simulink model "MicrochipTargetMotorControl"  (R2024b)
settings: Solver=FixedStepDiscrete  StartTime=0.0  StopTime=50  RelTol=1e-3  EnableMultiTasking=on
InitFcn:
  | MicrochipTargetMotorControlData;
  | mcbMotorSwapData;
values from neighbouring files (symbols this model uses):
  Ts = T_pwm    [mcbMotorSwapData.m]
  Ts_motor = T_pwm/2    [mcbMotorSwapData.m]
  Ts_serialIn = 50e-3    (= 0.05)    [MicrochipTargetMotorControlData.m]
  Ts_speed = 10*Ts    [mcbMotorSwapData.m]
undefined symbols (not defined in the file or in its folder): A4, B0, C10, C11, C6, C7, C8, inverter, MaxPer, P17, P20, P39, P40, P41, P43, P44, Pin, pmsm, Resol, s, target, Timer, us
libraries: MCHP_Blockset x19, simulink x13, autolibpmsminterior x1, mcbplantlib x1, mcbcontrolslib x1
(part 3 of 4)

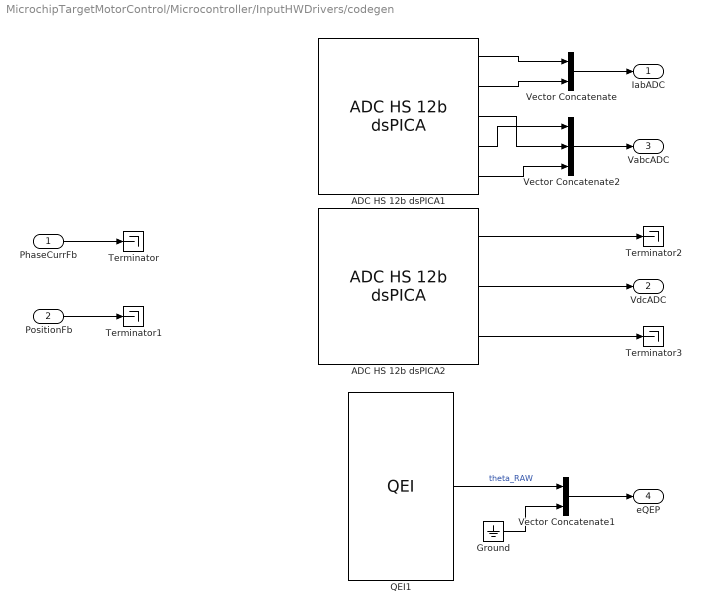
== system MicrochipTargetMotorControl/Microcontroller/InputHWDrivers/codegen ==
  PhaseCurrFb : Inport
  PositionFb : Inport  Port=2
  ADC HS 12b dsPICA1 : MCHP_Blockset/Analog IO/ADC HS 12b dsPICA  ADCREF=ADC 1 and ADC 2  ADC1_refChannel=0 (highest priority)  ADC2_refChannel=0 (highest priority)  ADC3_refChannel=Not used  ADC4_refChannel=Not used  ADC5_refChannel=Not used  CALRATE=once at startup  VREF_RNG=3.0V to 3.6V  BUFEN=off  info=0  SampleTime=Ts  MCHP_PORT={ADC1_seq0.0}{ADC1A2}15:2:A2;{ADC2_seq0.0}{ADC2B0}15:2:B0;{ADC1_seq0.1}{ADC1B8}15:2:B8;{ADC2_seq0.1}{ADC2B9}15:2:B9;{ADC2_seq0.2}{ADC2A10}15:2:A10;{ADC1_seq0.0}{ADC1A2}15:2:A2;{ADC2_seq0.0}{ADC2B0}15:2:B0;{ADC1_seq0.1}{ADC1B8}15:2:B8;{ADC2_seq0.1}{ADC2B9}15:2:B9;{ADC2_seq0.2}{ADC2A10}15:2:A10;  MCHP_MASTERLINK=MicrochipTargetMotorControl/Microcontroller/HWConfigurations/Microchip Master  MCHP_CRC=34200121  ADC_Synchronisation=Triggered by custom source  ADC_Trig_TXT=PWM1_Trg1  ADC_TrigTimeStep=on  TrigSource_seq0_TXT=PWM1 adc trig 0  SampleTime_seq0_Tad_TXT="4.5 Tad  = 56.2ns  -  Rin < 5.2 kOhm"  ADC1_seq0_TXT=AD1 AN0 / A2 / Pin[12]  ADC1_seq0_align=Right aligned  ADC1_seq0_overSampling=x1 (12 bits)  ADC2_seq0_TXT=AD2 AN1 / B0 / Pin[20]  ADC2_seq0_align=Right aligned  ADC2_seq0_overSampling=x1 (12 bits)  ADC3_seq0_TXT="AD2 AN1 / B0 / Pin[20]  (L)"  ADC3_seq0_align=Right aligned  ADC3_seq0_overSampling=x1 (12 bits)  ADC4_seq0_TXT="AD2 AN1 / B0 / Pin[20]  (L)"  ADC4_seq0_align=Right aligned  ADC4_seq0_overSampling=x1 (12 bits)  ADC5_seq0_TXT="AD2 AN1 / B0 / Pin[20]  (L)"  ADC5_seq0_align=Right aligned  ADC5_seq0_overSampling=x1 (12 bits)  ADC1_seq0_1_TXT=AD1 AN11 / B8 / Pin[23]  ADC1_seq0_1_align=Right aligned  ADC1_seq0_1_overSampling=x1 (12 bits)  ADC2_seq0_1_TXT=AD2 AN10 / B9 / Pin[24]  ADC2_seq0_1_align=Right aligned  ADC2_seq0_1_overSampling=x1 (12 bits)  ADC3_seq0_1_TXT=Not Used  ADC3_seq0_1_align=Right aligned  ADC3_seq0_1_overSampling=x1 (12 bits)  ADC4_seq0_1_TXT=Not Used  ADC4_seq0_1_align=Right aligned  ADC4_seq0_1_overSampling=x1 (12 bits)  ADC5_seq0_1_TXT=Not Used  ADC5_seq0_1_align=Right aligned  ADC5_seq0_1_overSampling=x1 (12 bits)  ADC1_seq0_2_TXT=Not Used  ADC1_seq0_2_align=Right aligned  ADC1_seq0_2_overSampling=x1 (12 bits)  ADC2_seq0_2_TXT=AD2 AN7 / A10 / Pin[9]  ADC2_seq0_2_align=Right aligned  ADC2_seq0_2_overSampling=x1 (12 bits)  ADC3_seq0_2_TXT=Not Used  ADC3_seq0_2_align=Right aligned  ADC3_seq0_2_overSampling=x1 (12 bits)  ADC4_seq0_2_TXT=Not Used  ADC4_seq0_2_align=Right aligned  ADC4_seq0_2_overSampling=x1 (12 bits)  ADC5_seq0_2_TXT=Not Used  ADC5_seq0_2_align=Right aligned  ADC5_seq0_2_overSampling=x1 (12 bits)  ADC1_seq0_3_TXT=Not Used  ADC1_seq0_3_align=Right aligned  ADC1_seq0_3_overSampling=x1 (12 bits)  ADC2_seq0_3_TXT=Not Used  ADC2_seq0_3_align=Right aligned  ADC2_seq0_3_overSampling=x1 (12 bits)  ADC3_seq0_3_TXT=Not Used  ADC3_seq0_3_align=Right aligned  ADC3_seq0_3_overSampling=x1 (12 bits)  ADC4_seq0_3_TXT=Not Used  ADC4_seq0_3_align=Right aligned  ADC4_seq0_3_overSampling=x1 (12 bits)  ADC5_seq0_3_TXT=Not Used  ADC5_seq0_3_align=Right aligned  ADC5_seq0_3_overSampling=x1 (12 bits)  ADC1_seq0_4_TXT=Not Used  ADC1_seq0_4_align=Right aligned  ADC1_seq0_4_overSampling=x1 (12 bits)  ADC2_seq0_4_TXT=Not Used  ADC2_seq0_4_align=Right aligned  ADC2_seq0_4_overSampling=x1 (12 bits)  ADC3_seq0_4_TXT=Not Used  ADC3_seq0_4_align=Right aligned  ADC3_seq0_4_overSampling=x1 (12 bits)  ADC4_seq0_4_TXT=Not Used  ADC4_seq0_4_align=Right aligned  ADC4_seq0_4_overSampling=x1 (12 bits)  ADC5_seq0_4_TXT=Not Used  ADC5_seq0_4_align=Right aligned  ADC5_seq0_4_overSampling=x1 (12 bits)  ADC1_seq0_5_TXT=Not Used  ADC1_seq0_5_align=Right aligned  ADC1_seq0_5_overSampling=x1 (12 bits)  ADC2_seq0_5_TXT=Not Used  ADC2_seq0_5_align=Right aligned  ADC2_seq0_5_overSampling=x1 (12 bits)  ADC3_seq0_5_TXT=Not Used  ADC3_seq0_5_align=Right aligned  ADC3_seq0_5_overSampling=x1 (12 bits)  ADC4_seq0_5_TXT=Not Used  ADC4_seq0_5_align=Right aligned  ADC4_seq0_5_overSampling=x1 (12 bits)  ADC5_seq0_5_TXT=Not Used  ADC5_seq0_5_align=Right aligned  ADC5_seq0_5_overSampling=x1 (12 bits)  ADC_TRG2_ACCBRST_seq0=Burst - not interruptible  ADC1_NINSEL_seq0_TXT=Vss - single ended (unsigned)  ADC2_NINSEL_seq0_TXT=Vss - single ended (unsigned)  ADC3_NINSEL_seq0_TXT=Vss - single ended (unsigned)  ADC4_NINSEL_seq0_TXT=Vss - single ended (unsigned)  ADC5_NINSEL_seq0_TXT=Vss - single ended (unsigned)  TrigTimeStep_seq0=on  info_seq0=0  TrigSource_seq1_TXT=after previous sequence  SampleTime_seq1_Tad_TXT="0.5 Tad  = 6.25ns  -  Rin < 0 kOhm"  ADC1_seq1_TXT=Not Used  ADC1_seq1_align=Right aligned  ADC1_seq1_overSampling=x1 (12 bits)  ADC2_seq1_TXT=Not Used  ADC2_seq1_align=Right aligned  ADC2_seq1_overSampling=x1 (12 bits)  ADC3_seq1_TXT=Not Used  ADC3_seq1_align=Right aligned  ADC3_seq1_overSampling=x1 (12 bits)  ADC4_seq1_TXT=Not Used  ADC4_seq1_align=Right aligned  ADC4_seq1_overSampling=x1 (12 bits)  ADC5_seq1_TXT=Not Used  ADC5_seq1_align=Right aligned  ADC5_seq1_overSampling=x1 (12 bits)  ADC1_seq1_1_TXT=Not Used  ADC1_seq1_1_align=Right aligned  ADC1_seq1_1_overSampling=x1 (12 bits)  ADC2_seq1_1_TXT=Not Used  ADC2_seq1_1_align=Right aligned  ADC2_seq1_1_overSampling=x1 (12 bits)  ADC3_seq1_1_TXT=Not Used  ADC3_seq1_1_align=Right aligned  ADC3_seq1_1_overSampling=x1 (12 bits)  ADC4_seq1_1_TXT=Not Used  ADC4_seq1_1_align=Right aligned  ADC4_seq1_1_overSampling=x1 (12 bits)  ADC5_seq1_1_TXT=Not Used  ADC5_seq1_1_align=Right aligned  ADC5_seq1_1_overSampling=x1 (12 bits)  ADC1_seq1_2_TXT=Not Used  ADC1_seq1_2_align=Right aligned  ADC1_seq1_2_overSampling=x1 (12 bits)  ADC2_seq1_2_TXT=Not Used  ADC2_seq1_2_align=Right aligned  ADC2_seq1_2_overSampling=x1 (12 bits)  ADC3_seq1_2_TXT=Not Used  ADC3_seq1_2_align=Right aligned  ADC3_seq1_2_overSampling=x1 (12 bits)  ADC4_seq1_2_TXT=Not Used  ADC4_seq1_2_align=Right aligned  ADC4_seq1_2_overSampling=x1 (12 bits)  ADC5_seq1_2_TXT=Not Used  ADC5_seq1_2_align=Right aligned  ADC5_seq1_2_overSampling=x1 (12 bits)  ADC1_seq1_3_TXT=Not Used  ADC1_seq1_3_align=Right aligned  ADC1_seq1_3_overSampling=x1 (12 bits)  ADC2_seq1_3_TXT=Not Used  ADC2_seq1_3_align=Right aligned  ADC2_seq1_3_overSampling=x1 (12 bits)  ADC3_seq1_3_TXT=Not Used  ADC3_seq1_3_align=Right aligned  ADC3_seq1_3_overSampling=x1 (12 bits)  ADC4_seq1_3_TXT=Not Used  ADC4_seq1_3_align=Right aligned  ADC4_seq1_3_overSampling=x1 (12 bits)  ADC5_seq1_3_TXT=Not Used  ADC5_seq1_3_align=Right aligned  ADC5_seq1_3_overSampling=x1 (12 bits)  ADC1_seq1_4_TXT=Not Used  ADC1_seq1_4_align=Right aligned  ADC1_seq1_4_overSampling=x1 (12 bits)  ADC2_seq1_4_TXT=Not Used  ADC2_seq1_4_align=Right aligned  ADC2_seq1_4_overSampling=x1 (12 bits)  ADC3_seq1_4_TXT=Not Used  ADC3_seq1_4_align=Right aligned  ADC3_seq1_4_overSampling=x1 (12 bits)  ADC4_seq1_4_TXT=Not Used  ADC4_seq1_4_align=Right aligned  ADC4_seq1_4_overSampling=x1 (12 bits)  ADC5_seq1_4_TXT=Not Used  ADC5_seq1_4_align=Right aligned  ADC5_seq1_4_overSampling=x1 (12 bits)  ADC1_seq1_5_TXT=Not Used  ADC1_seq1_5_align=Right aligned  ADC1_seq1_5_overSampling=x1 (12 bits)  ADC2_seq1_5_TXT=Not Used  ADC2_seq1_5_align=Right aligned  ADC2_seq1_5_overSampling=x1 (12 bits)  ADC3_seq1_5_TXT=Not Used  ADC3_seq1_5_align=Right aligned  ADC3_seq1_5_overSampling=x1 (12 bits)  ADC4_seq1_5_TXT=Not Used  ADC4_seq1_5_align=Right aligned  ADC4_seq1_5_overSampling=x1 (12 bits)  ADC5_seq1_5_TXT=Not Used  ADC5_seq1_5_align=Right aligned  ADC5_seq1_5_overSampling=x1 (12 bits)  ADC_TRG2_ACCBRST_seq1=Burst - not interruptible  ADC1_NINSEL_seq1_TXT=Vss - single ended (unsigned)  ADC2_NINSEL_seq1_TXT=Vss - single ended (unsigned)  ADC3_NINSEL_seq1_TXT=Vss - single ended (unsigned)  ADC4_NINSEL_seq1_TXT=Vss - single ended (unsigned)  ADC5_NINSEL_seq1_TXT=Vss - single ended (unsigned)  TrigTimeStep_seq1=off  info_seq1=0  TrigSource_seq2_TXT=after previous sequence  SampleTime_seq2_Tad_TXT="0.5 Tad  = 6.25ns  -  Rin < 0 kOhm"  ADC1_seq2_TXT=Not Used  ADC1_seq2_align=Right aligned  ADC1_seq2_overSampling=x1 (12 bits)  ADC2_seq2_TXT=Not Used  ADC2_seq2_align=Right aligned  ADC2_seq2_overSampling=x1 (12 bits)  ADC3_seq2_TXT=Not Used  ADC3_seq2_align=Right aligned  ADC3_seq2_overSampling=x1 (12 bits)  ADC4_seq2_TXT=Not Used  ADC4_seq2_align=Right aligned  ADC4_seq2_overSampling=x1 (12 bits)  ADC5_seq2_TXT=Not Used  ADC5_seq2_align=Right aligned  ADC5_seq2_overSampling=x1 (12 bits)  ADC1_seq2_1_TXT=Not Used  ADC1_seq2_1_align=Right aligned  ADC1_seq2_1_overSampling=x1 (12 bits)  ADC2_seq2_1_TXT=Not Used  ADC2_seq2_1_align=Right aligned  ADC2_seq2_1_overSampling=x1 (12 bits)  ADC3_seq2_1_TXT=Not Used  ADC3_seq2_1_align=Right aligned  ADC3_seq2_1_overSampling=x1 (12 bits)  ADC4_seq2_1_TXT=Not Used  ADC4_seq2_1_align=Right aligned  ADC4_seq2_1_overSampling=x1 (12 bits)  ADC5_seq2_1_TXT=Not Used  ADC5_seq2_1_align=Right aligned  ADC5_seq2_1_overSampling=x1 (12 bits)  ADC1_seq2_2_TXT=Not Used  ADC1_seq2_2_align=Right aligned  ADC1_seq2_2_overSampling=x1 (12 bits)  ADC2_seq2_2_TXT=Not Used  ADC2_seq2_2_align=Right aligned  ADC2_seq2_2_overSampling=x1 (12 bits)  ADC3_seq2_2_TXT=Not Used  ADC3_seq2_2_align=Right aligned  ADC3_seq2_2_overSampling=x1 (12 bits)  ADC4_seq2_2_TXT=Not Used  ADC4_seq2_2_align=Right aligned  ADC4_seq2_2_overSampling=x1 (12 bits)  ADC5_seq2_2_TXT=Not Used  ADC5_seq2_2_align=Right aligned  ADC5_seq2_2_overSampling=x1 (12 bits)  ADC1_seq2_3_TXT=Not Used  ADC1_seq2_3_align=Right aligned  ADC1_seq2_3_overSampling=x1 (12 bits)  ADC2_seq2_3_TXT=Not Used  ADC2_seq2_3_align=Right aligned  ADC2_seq2_3_overSampling=x1 (12 bits)  ADC3_seq2_3_TXT=Not Used  ADC3_seq2_3_align=Right aligned  ADC3_seq2_3_overSampling=x1 (12 bits)  ADC4_seq2_3_TXT=Not Used  ADC4_seq2_3_align=Right aligned  ADC4_seq2_3_overSampling=x1 (12 bits)  ADC5_seq2_3_TXT=Not Used  ADC5_seq2_3_align=Right aligned  ADC5_seq2_3_overSampling=x1 (12 bits)  ADC1_seq2_4_TXT=Not Used  ADC1_seq2_4_align=Right aligned  ADC1_seq2_4_overSampling=x1 (12 bits)  ADC2_seq2_4_TXT=Not Used  ADC2_seq2_4_align=Right aligned  ADC2_seq2_4_overSampling=x1 (12 bits)  ADC3_seq2_4_TXT=Not Used  ADC3_seq2_4_align=Right aligned  ADC3_seq2_4_overSampling=x1 (12 bits)  ADC4_seq2_4_TXT=Not Used  ADC4_seq2_4_align=Right aligned  ADC4_seq2_4_overSampling=x1 (12 bits)  ADC5_seq2_4_TXT=Not Used  ADC5_seq2_4_align=Right aligned  ADC5_seq2_4_overSampling=x1 (12 bits)  ADC1_seq2_5_TXT=Not Used  ADC1_seq2_5_align=Right aligned  ADC1_seq2_5_overSampling=x1 (12 bits)  ADC2_seq2_5_TXT=Not Used  ADC2_seq2_5_align=Right aligned  ADC2_seq2_5_overSampling=x1 (12 bits)  ADC3_seq2_5_TXT=Not Used  ADC3_seq2_5_align=Right aligned  ADC3_seq2_5_overSampling=x1 (12 bits)  ADC4_seq2_5_TXT=Not Used  ADC4_seq2_5_align=Right aligned  ADC4_seq2_5_overSampling=x1 (12 bits)  ADC5_seq2_5_TXT=Not Used  ADC5_seq2_5_align=Right aligned  ADC5_seq2_5_overSampling=x1 (12 bits)  ADC_TRG2_ACCBRST_seq2=Burst - not interruptible  ADC1_NINSEL_seq2_TXT=Vss - single ended (unsigned)  ADC2_NINSEL_seq2_TXT=Vss - single ended (unsigned)  ADC3_NINSEL_seq2_TXT=Vss - single ended (unsigned)  ADC4_NINSEL_seq2_TXT=Vss - single ended (unsigned)  ADC5_NINSEL_seq2_TXT=Vss - single ended (unsigned)  TrigTimeStep_seq2=off  info_seq2=0  TrigSource_seq3_TXT=after previous sequence  SampleTime_seq3_Tad_TXT="0.5 Tad  = 6.25ns  -  Rin < 0 kOhm"  ADC1_seq3_TXT=Not Used  ADC1_seq3_align=Right aligned  ADC1_seq3_overSampling=x1 (12 bits)  ADC2_seq3_TXT=Not Used  ADC2_seq3_align=Right aligned  ADC2_seq3_overSampling=x1 (12 bits)  ADC3_seq3_TXT=Not Used  ADC3_seq3_align=Right aligned  ADC3_seq3_overSampling=x1 (12 bits)  ADC4_seq3_TXT=Not Used  ADC4_seq3_align=Right aligned  ADC4_seq3_overSampling=x1 (12 bits)  ADC5_seq3_TXT=Not Used  ADC5_seq3_align=Right aligned  ADC5_seq3_overSampling=x1 (12 bits)  ADC1_seq3_1_TXT=Not Used  ADC1_seq3_1_align=Right aligned  ADC1_seq3_1_overSampling=x1 (12 bits)  ADC2_seq3_1_TXT=Not Used  ADC2_seq3_1_align=Right aligned  ADC2_seq3_1_overSampling=x1 (12 bits)  ADC3_seq3_1_TXT=Not Used  ADC3_seq3_1_align=Right aligned  ADC3_seq3_1_overSampling=x1 (12 bits)  ADC4_seq3_1_TXT=Not Used  ADC4_seq3_1_align=Right aligned  ADC4_seq3_1_overSampling=x1 (12 bits)  ADC5_seq3_1_TXT=Not Used  ADC5_seq3_1_align=Right aligned  ADC5_seq3_1_overSampling=x1 (12 bits)  ADC1_seq3_2_TXT=Not Used  ADC1_seq3_2_align=Right aligned  ADC1_seq3_2_overSampling=x1 (12 bits)  ADC2_seq3_2_TXT=Not Used  ADC2_seq3_2_align=Right aligned  ADC2_seq3_2_overSampling=x1 (12 bits)  ADC3_seq3_2_TXT=Not Used  ADC3_seq3_2_align=Right aligned  ADC3_seq3_2_overSampling=x1 (12 bits)  ADC4_seq3_2_TXT=Not Used  ADC4_seq3_2_align=Right aligned  ADC4_seq3_2_overSampling=x1 (12 bits)  ADC5_seq3_2_TXT=Not Used  ADC5_seq3_2_align=Right aligned  ADC5_seq3_2_overSampling=x1 (12 bits)  ADC1_seq3_3_TXT=Not Used  ADC1_seq3_3_align=Right aligned  ADC1_seq3_3_overSampling=x1 (12 bits)  ADC2_seq3_3_TXT=Not Used  ADC2_seq3_3_align=Right aligned  ADC2_seq3_3_overSampling=x1 (12 bits)  ADC3_seq3_3_TXT=Not Used  ADC3_seq3_3_align=Right aligned  ADC3_seq3_3_overSampling=x1 (12 bits)  ADC4_seq3_3_TXT=Not Used  ADC4_seq3_3_align=Right aligned  ADC4_seq3_3_overSampling=x1 (12 bits)  ADC5_seq3_3_TXT=Not Used  ADC5_seq3_3_align=Right aligned  ADC5_seq3_3_overSampling=x1 (12 bits)  ADC1_seq3_4_TXT=Not Used  ADC1_seq3_4_align=Right aligned  ADC1_seq3_4_overSampling=x1 (12 bits)  ADC2_seq3_4_TXT=Not Used  ADC2_seq3_4_align=Right aligned  ADC2_seq3_4_overSampling=x1 (12 bits)  ADC3_seq3_4_TXT=Not Used  ADC3_seq3_4_align=Right aligned  ADC3_seq3_4_overSampling=x1 (12 bits)  ADC4_seq3_4_TXT=Not Used  ADC4_seq3_4_align=Right aligned  ADC4_seq3_4_overSampling=x1 (12 bits)  ADC5_seq3_4_TXT=Not Used  ADC5_seq3_4_align=Right aligned  ADC5_seq3_4_overSampling=x1 (12 bits)  ADC1_seq3_5_TXT=Not Used  ADC1_seq3_5_align=Right aligned  ADC1_seq3_5_overSampling=x1 (12 bits)  ADC2_seq3_5_TXT=Not Used  ADC2_seq3_5_align=Right aligned  ADC2_seq3_5_overSampling=x1 (12 bits)  ADC3_seq3_5_TXT=Not Used  ADC3_seq3_5_align=Right aligned  ADC3_seq3_5_overSampling=x1 (12 bits)  ADC4_seq3_5_TXT=Not Used  ADC4_seq3_5_align=Right aligned  ADC4_seq3_5_overSampling=x1 (12 bits)  ADC5_seq3_5_TXT=Not Used  ADC5_seq3_5_align=Right aligned  ADC5_seq3_5_overSampling=x1 (12 bits)  ADC_TRG2_ACCBRST_seq3=Burst - not interruptible  ADC1_NINSEL_seq3_TXT=Vss - single ended (unsigned)  ADC2_NINSEL_seq3_TXT=Vss - single ended (unsigned)  ADC3_NINSEL_seq3_TXT=Vss - single ended (unsigned)  ADC4_NINSEL_seq3_TXT=Vss - single ended (unsigned)  ADC5_NINSEL_seq3_TXT=Vss - single ended (unsigned)  TrigTimeStep_seq3=off  info_seq3=0  TrigSource_seq4_TXT=after previous sequence  SampleTime_seq4_Tad_TXT="0.5 Tad  = 6.25ns  -  Rin < 0 kOhm"  ADC1_seq4_TXT=Not Used  ADC1_seq4_align=Right aligned  ADC1_seq4_overSampling=x1 (12 bits)  ADC2_seq4_TXT=Not Used  ADC2_seq4_align=Right aligned  ADC2_seq4_overSampling=x1 (12 bits)  ADC3_seq4_TXT=Not Used  ADC3_seq4_align=Right aligned  ADC3_seq4_overSampling=x1 (12 bits)  ADC4_seq4_TXT=Not Used  ADC4_seq4_align=Right aligned  ADC4_seq4_overSampling=x1 (12 bits)  ADC5_seq4_TXT=Not Used  ADC5_seq4_align=Right aligned  ADC5_seq4_overSampling=x1 (12 bits)  ADC1_seq4_1_TXT=Not Used  ADC1_seq4_1_align=Right aligned  ADC1_seq4_1_overSampling=x1 (12 bits)  ADC2_seq4_1_TXT=Not Used  ADC2_seq4_1_align=Right aligned  ADC2_seq4_1_overSampling=x1 (12 bits)  ADC3_seq4_1_TXT=Not Used  ADC3_seq4_1_align=Right aligned  ADC3_seq4_1_overSampling=x1 (12 bits)  ADC4_seq4_1_TXT=Not Used  ADC4_seq4_1_align=Right aligned  ADC4_seq4_1_overSampling=x1 (12 bits)  ADC5_seq4_1_TXT=Not Used  ADC5_seq4_1_align=Right aligned  ADC5_seq4_1_overSampling=x1 (12 bits)  ADC1_seq4_2_TXT=Not Used  ADC1_seq4_2_align=Right aligned  ADC1_seq4_2_overSampling=x1 (12 bits)  ADC2_seq4_2_TXT=Not Used  ADC2_seq4_2_align=Right aligned  ADC2_seq4_2_overSampling=x1 (12 bits)  ADC3_seq4_2_TXT=Not Used  ADC3_seq4_2_align=Right aligned  ADC3_seq4_2_overSampling=x1 (12 bits)  ADC4_seq4_2_TXT=Not Used  ADC4_seq4_2_align=Right aligned  ADC4_seq4_2_overSampling=x1 (12 bits)  ADC5_seq4_2_TXT=Not Used  ADC5_seq4_2_align=Right aligned  ADC5_seq4_2_overSampling=x1 (12 bits)  ADC1_seq4_3_TXT=Not Used  ADC1_seq4_3_align=Right aligned  ADC1_seq4_3_overSampling=x1 (12 bits)  ADC2_seq4_3_TXT=Not Used  ADC2_seq4_3_align=Right aligned  ADC2_seq4_3_overSampling=x1 (12 bits)  ADC3_seq4_3_TXT=Not Used  ADC3_seq4_3_align=Right aligned  ADC3_seq4_3_overSampling=x1 (12 bits)  ADC4_seq4_3_TXT=Not Used  ADC4_seq4_3_align=Right aligned  ADC4_seq4_3_overSampling=x1 (12 bits)  ADC5_seq4_3_TXT=Not Used  ADC5_seq4_3_align=Right aligned  ADC5_seq4_3_overSampling=x1 (12 bits)  ADC1_seq4_4_TXT=Not Used  ADC1_seq4_4_align=Right aligned  ADC1_seq4_4_overSampling=x1 (12 bits)  ADC2_seq4_4_TXT=Not Used  ADC2_seq4_4_align=Right aligned  ADC2_seq4_4_overSampling=x1 (12 bits)  ADC3_seq4_4_TXT=Not Used  ADC3_seq4_4_align=Right aligned  ADC3_seq4_4_overSampling=x1 (12 bits)  ADC4_seq4_4_TXT=Not Used  ADC4_seq4_4_align=Right aligned  ADC4_seq4_4_overSampling=x1 (12 bits)  ADC5_seq4_4_TXT=Not Used  ADC5_seq4_4_align=Right aligned  ADC5_seq4_4_overSampling=x1 (12 bits)  ADC1_seq4_5_TXT=Not Used  ADC1_seq4_5_align=Right aligned  ADC1_seq4_5_overSampling=x1 (12 bits)  ADC2_seq4_5_TXT=Not Used  ADC2_seq4_5_align=Right aligned  ADC2_seq4_5_overSampling=x1 (12 bits)  ADC3_seq4_5_TXT=Not Used  ADC3_seq4_5_align=Right aligned  ADC3_seq4_5_overSampling=x1 (12 bits)  ADC4_seq4_5_TXT=Not Used  ADC4_seq4_5_align=Right aligned  ADC4_seq4_5_overSampling=x1 (12 bits)  ADC5_seq4_5_TXT=Not Used  ADC5_seq4_5_align=Right aligned  ADC5_seq4_5_overSampling=x1 (12 bits)  ADC_TRG2_ACCBRST_seq4=Burst - not interruptible  ADC1_NINSEL_seq4_TXT=Vss - single ended (unsigned)  ADC2_NINSEL_seq4_TXT=Vss - single ended (unsigned)  ADC3_NINSEL_seq4_TXT=Vss - single ended (unsigned)  ADC4_NINSEL_seq4_TXT=Vss - single ended (unsigned)  ADC5_NINSEL_seq4_TXT=Vss - single ended (unsigned)  TrigTimeStep_seq4=off  info_seq4=0  TrigSource_seq5_TXT=after previous sequence  SampleTime_seq5_Tad_TXT="0.5 Tad  = 6.25ns  -  Rin < 0 kOhm"  ADC1_seq5_TXT=Not Used  ADC1_seq5_align=Right aligned  ADC1_seq5_overSampling=x1 (12 bits)  ADC2_seq5_TXT=Not Used  ADC2_seq5_align=Right aligned  ADC2_seq5_overSampling=x1 (12 bits)  ADC3_seq5_TXT=Not Used  ADC3_seq5_align=Right aligned  ADC3_seq5_overSampling=x1 (12 bits)  ADC4_seq5_TXT=Not Used  ADC4_seq5_align=Right aligned  ADC4_seq5_overSampling=x1 (12 bits)  ADC5_seq5_TXT=Not Used  ADC5_seq5_align=Right aligned  ADC5_seq5_overSampling=x1 (12 bits)  ADC1_seq5_1_TXT=Not Used  ADC1_seq5_1_align=Right aligned  ADC1_seq5_1_overSampling=x1 (12 bits)  ADC2_seq5_1_TXT=Not Used  ADC2_seq5_1_align=Right aligned  ADC2_seq5_1_overSampling=x1 (12 bits)  ADC3_seq5_1_TXT=Not Used  ADC3_seq5_1_align=Right aligned  ADC3_seq5_1_overSampling=x1 (12 bits)  ADC4_seq5_1_TXT=Not Used  ADC4_seq5_1_align=Right aligned  ADC4_seq5_1_overSampling=x1 (12 bits)  ADC5_seq5_1_TXT=Not Used  ADC5_seq5_1_align=Right aligned  ADC5_seq5_1_overSampling=x1 (12 bits)  ADC1_seq5_2_TXT=Not Used  ADC1_seq5_2_align=Right aligned  ADC1_seq5_2_overSampling=x1 (12 bits)  ADC2_seq5_2_TXT=Not Used  ADC2_seq5_2_align=Right aligned  ADC2_seq5_2_overSampling=x1 (12 bits)  ADC3_seq5_2_TXT=Not Used  ADC3_seq5_2_align=Right aligned  ADC3_seq5_2_overSampling=x1 (12 bits)  ADC4_seq5_2_TXT=Not Used  ADC4_seq5_2_align=Right aligned  ADC4_seq5_2_overSampling=x1 (12 bits)  ADC5_seq5_2_TXT=Not Used  ADC5_seq5_2_align=Right aligned  ADC5_seq5_2_overSampling=x1 (12 bits)  ADC1_seq5_3_TXT=Not Used  ADC1_seq5_3_align=Right aligned  ADC1_seq5_3_overSampling=x1 (12 bits)  ADC2_seq5_3_TXT=Not Used  ADC2_seq5_3_align=Right aligned  ADC2_seq5_3_overSampling=x1 (12 bits)  ADC3_seq5_3_TXT=Not Used  ADC3_seq5_3_align=Right aligned  ADC3_seq5_3_overSampling=x1 (12 bits)  ADC4_seq5_3_TXT=Not Used  ADC4_seq5_3_align=Right aligned  ADC4_seq5_3_overSampling=x1 (12 bits)  ADC5_seq5_3_TXT=Not Used  ADC5_seq5_3_align=Right aligned  ADC5_seq5_3_overSampling=x1 (12 bits)  ADC1_seq5_4_TXT=Not Used  ADC1_seq5_4_align=Right aligned  ADC1_seq5_4_overSampling=x1 (12 bits)  ADC2_seq5_4_TXT=Not Used  ADC2_seq5_4_align=Right aligned  ADC2_seq5_4_overSampling=x1 (12 bits)  ADC3_seq5_4_TXT=Not Used  ADC3_seq5_4_align=Right aligned  ADC3_seq5_4_overSampling=x1 (12 bits)  ADC4_seq5_4_TXT=Not Used  ADC4_seq5_4_align=Right aligned  ADC4_seq5_4_overSampling=x1 (12 bits)  ADC5_seq5_4_TXT=Not Used  ADC5_seq5_4_align=Right aligned  ADC5_seq5_4_overSampling=x1 (12 bits)  ADC1_seq5_5_TXT=Not Used  ADC1_seq5_5_align=Right aligned  ADC1_seq5_5_overSampling=x1 (12 bits)  ADC2_seq5_5_TXT=Not Used  ADC2_seq5_5_align=Right aligned  ADC2_seq5_5_overSampling=x1 (12 bits)  ADC3_seq5_5_TXT=Not Used  ADC3_seq5_5_align=Right aligned  ADC3_seq5_5_overSampling=x1 (12 bits)  ADC4_seq5_5_TXT=Not Used  ADC4_seq5_5_align=Right aligned  ADC4_seq5_5_overSampling=x1 (12 bits)  ADC5_seq5_5_TXT=Not Used  ADC5_seq5_5_align=Right aligned  ADC5_seq5_5_overSampling=x1 (12 bits)  ADC_TRG2_ACCBRST_seq5=Burst - not interruptible  ADC1_NINSEL_seq5_TXT=Vss - single ended (unsigned)  ADC2_NINSEL_seq5_TXT=Vss - single ended (unsigned)  ADC3_NINSEL_seq5_TXT=Vss - single ended (unsigned)  ADC4_NINSEL_seq5_TXT=Vss - single ended (unsigned)  ADC5_NINSEL_seq5_TXT=Vss - single ended (unsigned)  TrigTimeStep_seq5=off  info_seq5=0
      settings: SourceProductName=MPLAB Device Blocks for Simulink
  ADC HS 12b dsPICA2 : MCHP_Blockset/Analog IO/ADC HS 12b dsPICA  ADCREF=ADC 1  ADC1_refChannel=5  ADC2_refChannel=5  ADC3_refChannel=Not used  ADC4_refChannel=Not used  ADC5_refChannel=Not used  CALRATE=once at startup  VREF_RNG=3.0V to 3.6V  BUFEN=off  info=0  SampleTime=Ts  MCHP_PORT={ADC1_seq0.0}{ADC1A5}15:2:A5;{ADC1_seq0.1}{ADC1A7}15:2:A7;{ADC1_seq0.2}{ADC1A11}15:2:A11;{ADC1_seq0.0}{ADC1A5}15:2:A5;{ADC1_seq0.1}{ADC1A7}15:2:A7;{ADC1_seq0.2}{ADC1A11}15:2:A11;  MCHP_MASTERLINK=MicrochipTargetMotorControl/Microcontroller/HWConfigurations/Microchip Master  MCHP_CRC=34100181  ADC_Synchronisation=off  ADC_Trig_TXT=off  ADC_TrigTimeStep=off  TrigSource_seq0_TXT=PWM1 adc trig 0  SampleTime_seq0_Tad_TXT="8.5 Tad  = 106ns  -  Rin < 11 kOhm"  ADC1_seq0_TXT=AD1 AN3 / A5 / Pin[15]  ADC1_seq0_align=Right aligned  ADC1_seq0_overSampling=x1 (12 bits)  ADC2_seq0_TXT=Not Used  ADC2_seq0_align=Right aligned  ADC2_seq0_overSampling=x1 (12 bits)  ADC3_seq0_TXT="AD2 AN1 / B0 / Pin[20]  (L)"  ADC3_seq0_align=Right aligned  ADC3_seq0_overSampling=x1 (12 bits)  ADC4_seq0_TXT="AD2 AN1 / B0 / Pin[20]  (L)"  ADC4_seq0_align=Right aligned  ADC4_seq0_overSampling=x1 (12 bits)  ADC5_seq0_TXT="AD2 AN1 / B0 / Pin[20]  (L)"  ADC5_seq0_align=Right aligned  ADC5_seq0_overSampling=x1 (12 bits)  ADC1_seq0_1_TXT=AD1 AN6 / A7 / Pin[2]  ADC1_seq0_1_align=Right aligned  ADC1_seq0_1_overSampling=x1 (12 bits)  ADC2_seq0_1_TXT=Not Used  ADC2_seq0_1_align=Right aligned  ADC2_seq0_1_overSampling=x1 (12 bits)  ADC3_seq0_1_TXT=Not Used  ADC3_seq0_1_align=Right aligned  ADC3_seq0_1_overSampling=x1 (12 bits)  ADC4_seq0_1_TXT=Not Used  ADC4_seq0_1_align=Right aligned  ADC4_seq0_1_overSampling=x1 (12 bits)  ADC5_seq0_1_TXT=Not Used  ADC5_seq0_1_align=Right aligned  ADC5_seq0_1_overSampling=x1 (12 bits)  ADC1_seq0_2_TXT=AD1 AN10 / A11 / Pin[6]  ADC1_seq0_2_align=Right aligned  ADC1_seq0_2_overSampling=x1 (12 bits)  ADC2_seq0_2_TXT=Not Used  ADC2_seq0_2_align=Right aligned  ADC2_seq0_2_overSampling=x1 (12 bits)  ADC3_seq0_2_TXT=Not Used  ADC3_seq0_2_align=Right aligned  ADC3_seq0_2_overSampling=x1 (12 bits)  ADC4_seq0_2_TXT=Not Used  ADC4_seq0_2_align=Right aligned  ADC4_seq0_2_overSampling=x1 (12 bits)  ADC5_seq0_2_TXT=Not Used  ADC5_seq0_2_align=Right aligned  ADC5_seq0_2_overSampling=x1 (12 bits)  ADC1_seq0_3_TXT=Not Used  ADC1_seq0_3_align=Right aligned  ADC1_seq0_3_overSampling=x1 (12 bits)  ADC2_seq0_3_TXT=Not Used  ADC2_seq0_3_align=Right aligned  ADC2_seq0_3_overSampling=x1 (12 bits)  ADC3_seq0_3_TXT=Not Used  ADC3_seq0_3_align=Right aligned  ADC3_seq0_3_overSampling=x1 (12 bits)  ADC4_seq0_3_TXT=Not Used  ADC4_seq0_3_align=Right aligned  ADC4_seq0_3_overSampling=x1 (12 bits)  ADC5_seq0_3_TXT=Not Used  ADC5_seq0_3_align=Right aligned  ADC5_seq0_3_overSampling=x1 (12 bits)  ADC1_seq0_4_TXT=Not Used  ADC1_seq0_4_align=Right aligned  ADC1_seq0_4_overSampling=x1 (12 bits)  ADC2_seq0_4_TXT=Not Used  ADC2_seq0_4_align=Right aligned  ADC2_seq0_4_overSampling=x1 (12 bits)  ADC3_seq0_4_TXT=Not Used  ADC3_seq0_4_align=Right aligned  ADC3_seq0_4_overSampling=x1 (12 bits)  ADC4_seq0_4_TXT=Not Used  ADC4_seq0_4_align=Right aligned  ADC4_seq0_4_overSampling=x1 (12 bits)  ADC5_seq0_4_TXT=Not Used  ADC5_seq0_4_align=Right aligned  ADC5_seq0_4_overSampling=x1 (12 bits)  ADC1_seq0_5_TXT=Not Used  ADC1_seq0_5_align=Right aligned  ADC1_seq0_5_overSampling=x1 (12 bits)  ADC2_seq0_5_TXT=Not Used  ADC2_seq0_5_align=Right aligned  ADC2_seq0_5_overSampling=x1 (12 bits)  ADC3_seq0_5_TXT=Not Used  ADC3_seq0_5_align=Right aligned  ADC3_seq0_5_overSampling=x1 (12 bits)  ADC4_seq0_5_TXT=Not Used  ADC4_seq0_5_align=Right aligned  ADC4_seq0_5_overSampling=x1 (12 bits)  ADC5_seq0_5_TXT=Not Used  ADC5_seq0_5_align=Right aligned  ADC5_seq0_5_overSampling=x1 (12 bits)  ADC_TRG2_ACCBRST_seq0=Burst - not interruptible  ADC1_NINSEL_seq0_TXT=Vss - single ended (unsigned)  ADC2_NINSEL_seq0_TXT=Vss - single ended (unsigned)  ADC3_NINSEL_seq0_TXT=Vss - single ended (unsigned)  ADC4_NINSEL_seq0_TXT=Vss - single ended (unsigned)  ADC5_NINSEL_seq0_TXT=Vss - single ended (unsigned)  TrigTimeStep_seq0=off  info_seq0=0  TrigSource_seq1_TXT=after previous sequence  SampleTime_seq1_Tad_TXT="0.5 Tad  = 6.25ns  -  Rin < 0 kOhm"  ADC1_seq1_TXT=Not Used  ADC1_seq1_align=Right aligned  ADC1_seq1_overSampling=x1 (12 bits)  ADC2_seq1_TXT=Not Used  ADC2_seq1_align=Right aligned  ADC2_seq1_overSampling=x1 (12 bits)  ADC3_seq1_TXT=Not Used  ADC3_seq1_align=Right aligned  ADC3_seq1_overSampling=x1 (12 bits)  ADC4_seq1_TXT=Not Used  ADC4_seq1_align=Right aligned  ADC4_seq1_overSampling=x1 (12 bits)  ADC5_seq1_TXT=Not Used  ADC5_seq1_align=Right aligned  ADC5_seq1_overSampling=x1 (12 bits)  ADC1_seq1_1_TXT=Not Used  ADC1_seq1_1_align=Right aligned  ADC1_seq1_1_overSampling=x1 (12 bits)  ADC2_seq1_1_TXT=Not Used  ADC2_seq1_1_align=Right aligned  ADC2_seq1_1_overSampling=x1 (12 bits)  ADC3_seq1_1_TXT=Not Used  ADC3_seq1_1_align=Right aligned  ADC3_seq1_1_overSampling=x1 (12 bits)  ADC4_seq1_1_TXT=Not Used  ADC4_seq1_1_align=Right aligned  ADC4_seq1_1_overSampling=x1 (12 bits)  ADC5_seq1_1_TXT=Not Used  ADC5_seq1_1_align=Right aligned  ADC5_seq1_1_overSampling=x1 (12 bits)  ADC1_seq1_2_TXT=Not Used  ADC1_seq1_2_align=Right aligned  ADC1_seq1_2_overSampling=x1 (12 bits)  ADC2_seq1_2_TXT=Not Used  ADC2_seq1_2_align=Right aligned  ADC2_seq1_2_overSampling=x1 (12 bits)  ADC3_seq1_2_TXT=Not Used  ADC3_seq1_2_align=Right aligned  ADC3_seq1_2_overSampling=x1 (12 bits)  ADC4_seq1_2_TXT=Not Used  ADC4_seq1_2_align=Right aligned  ADC4_seq1_2_overSampling=x1 (12 bits)  ADC5_seq1_2_TXT=Not Used  ADC5_seq1_2_align=Right aligned  ADC5_seq1_2_overSampling=x1 (12 bits)  ADC1_seq1_3_TXT=Not Used  ADC1_seq1_3_align=Right aligned  ADC1_seq1_3_overSampling=x1 (12 bits)  ADC2_seq1_3_TXT=Not Used  ADC2_seq1_3_align=Right aligned  ADC2_seq1_3_overSampling=x1 (12 bits)  ADC3_seq1_3_TXT=Not Used  ADC3_seq1_3_align=Right aligned  ADC3_seq1_3_overSampling=x1 (12 bits)  ADC4_seq1_3_TXT=Not Used  ADC4_seq1_3_align=Right aligned  ADC4_seq1_3_overSampling=x1 (12 bits)  ADC5_seq1_3_TXT=Not Used  ADC5_seq1_3_align=Right aligned  ADC5_seq1_3_overSampling=x1 (12 bits)  ADC1_seq1_4_TXT=Not Used  ADC1_seq1_4_align=Right aligned  ADC1_seq1_4_overSampling=x1 (12 bits)  ADC2_seq1_4_TXT=Not Used  ADC2_seq1_4_align=Right aligned  ADC2_seq1_4_overSampling=x1 (12 bits)  ADC3_seq1_4_TXT=Not Used  ADC3_seq1_4_align=Right aligned  ADC3_seq1_4_overSampling=x1 (12 bits)  ADC4_seq1_4_TXT=Not Used  ADC4_seq1_4_align=Right aligned  ADC4_seq1_4_overSampling=x1 (12 bits)  ADC5_seq1_4_TXT=Not Used  ADC5_seq1_4_align=Right aligned  ADC5_seq1_4_overSampling=x1 (12 bits)  ADC1_seq1_5_TXT=Not Used  ADC1_seq1_5_align=Right aligned  ADC1_seq1_5_overSampling=x1 (12 bits)  ADC2_seq1_5_TXT=Not Used  ADC2_seq1_5_align=Right aligned  ADC2_seq1_5_overSampling=x1 (12 bits)  ADC3_seq1_5_TXT=Not Used  ADC3_seq1_5_align=Right aligned  ADC3_seq1_5_overSampling=x1 (12 bits)  ADC4_seq1_5_TXT=Not Used  ADC4_seq1_5_align=Right aligned  ADC4_seq1_5_overSampling=x1 (12 bits)  ADC5_seq1_5_TXT=Not Used  ADC5_seq1_5_align=Right aligned  ADC5_seq1_5_overSampling=x1 (12 bits)  ADC_TRG2_ACCBRST_seq1=Burst - not interruptible  ADC1_NINSEL_seq1_TXT=Vss - single ended (unsigned)  ADC2_NINSEL_seq1_TXT=Vss - single ended (unsigned)  ADC3_NINSEL_seq1_TXT=Vss - single ended (unsigned)  ADC4_NINSEL_seq1_TXT=Vss - single ended (unsigned)  ADC5_NINSEL_seq1_TXT=Vss - single ended (unsigned)  TrigTimeStep_seq1=off  info_seq1=0  TrigSource_seq2_TXT=after previous sequence  SampleTime_seq2_Tad_TXT="0.5 Tad  = 6.25ns  -  Rin < 0 kOhm"  ADC1_seq2_TXT=Not Used  ADC1_seq2_align=Right aligned  ADC1_seq2_overSampling=x1 (12 bits)  ADC2_seq2_TXT=Not Used  ADC2_seq2_align=Right aligned  ADC2_seq2_overSampling=x1 (12 bits)  ADC3_seq2_TXT=Not Used  ADC3_seq2_align=Right aligned  ADC3_seq2_overSampling=x1 (12 bits)  ADC4_seq2_TXT=Not Used  ADC4_seq2_align=Right aligned  ADC4_seq2_overSampling=x1 (12 bits)  ADC5_seq2_TXT=Not Used  ADC5_seq2_align=Right aligned  ADC5_seq2_overSampling=x1 (12 bits)  ADC1_seq2_1_TXT=Not Used  ADC1_seq2_1_align=Right aligned  ADC1_seq2_1_overSampling=x1 (12 bits)  ADC2_seq2_1_TXT=Not Used  ADC2_seq2_1_align=Right aligned  ADC2_seq2_1_overSampling=x1 (12 bits)  ADC3_seq2_1_TXT=Not Used  ADC3_seq2_1_align=Right aligned  ADC3_seq2_1_overSampling=x1 (12 bits)  ADC4_seq2_1_TXT=Not Used  ADC4_seq2_1_align=Right aligned  ADC4_seq2_1_overSampling=x1 (12 bits)  ADC5_seq2_1_TXT=Not Used  ADC5_seq2_1_align=Right aligned  ADC5_seq2_1_overSampling=x1 (12 bits)  ADC1_seq2_2_TXT=Not Used  ADC1_seq2_2_align=Right aligned  ADC1_seq2_2_overSampling=x1 (12 bits)  ADC2_seq2_2_TXT=Not Used  ADC2_seq2_2_align=Right aligned  ADC2_seq2_2_overSampling=x1 (12 bits)  ADC3_seq2_2_TXT=Not Used  ADC3_seq2_2_align=Right aligned  ADC3_seq2_2_overSampling=x1 (12 bits)  ADC4_seq2_2_TXT=Not Used  ADC4_seq2_2_align=Right aligned  ADC4_seq2_2_overSampling=x1 (12 bits)  ADC5_seq2_2_TXT=Not Used  ADC5_seq2_2_align=Right aligned  ADC5_seq2_2_overSampling=x1 (12 bits)  ADC1_seq2_3_TXT=Not Used  ADC1_seq2_3_align=Right aligned  ADC1_seq2_3_overSampling=x1 (12 bits)  ADC2_seq2_3_TXT=Not Used  ADC2_seq2_3_align=Right aligned  ADC2_seq2_3_overSampling=x1 (12 bits)  ADC3_seq2_3_TXT=Not Used  ADC3_seq2_3_align=Right aligned  ADC3_seq2_3_overSampling=x1 (12 bits)  ADC4_seq2_3_TXT=Not Used  ADC4_seq2_3_align=Right aligned  ADC4_seq2_3_overSampling=x1 (12 bits)  ADC5_seq2_3_TXT=Not Used  ADC5_seq2_3_align=Right aligned  ADC5_seq2_3_overSampling=x1 (12 bits)  ADC1_seq2_4_TXT=Not Used  ADC1_seq2_4_align=Right aligned  ADC1_seq2_4_overSampling=x1 (12 bits)  ADC2_seq2_4_TXT=Not Used  ADC2_seq2_4_align=Right aligned  ADC2_seq2_4_overSampling=x1 (12 bits)  ADC3_seq2_4_TXT=Not Used  ADC3_seq2_4_align=Right aligned  ADC3_seq2_4_overSampling=x1 (12 bits)  ADC4_seq2_4_TXT=Not Used  ADC4_seq2_4_align=Right aligned  ADC4_seq2_4_overSampling=x1 (12 bits)  ADC5_seq2_4_TXT=Not Used  ADC5_seq2_4_align=Right aligned  ADC5_seq2_4_overSampling=x1 (12 bits)  ADC1_seq2_5_TXT=Not Used  ADC1_seq2_5_align=Right aligned  ADC1_seq2_5_overSampling=x1 (12 bits)  ADC2_seq2_5_TXT=Not Used  ADC2_seq2_5_align=Right aligned  ADC2_seq2_5_overSampling=x1 (12 bits)  ADC3_seq2_5_TXT=Not Used  ADC3_seq2_5_align=Right aligned  ADC3_seq2_5_overSampling=x1 (12 bits)  ADC4_seq2_5_TXT=Not Used  ADC4_seq2_5_align=Right aligned  ADC4_seq2_5_overSampling=x1 (12 bits)  ADC5_seq2_5_TXT=Not Used  ADC5_seq2_5_align=Right aligned  ADC5_seq2_5_overSampling=x1 (12 bits)  ADC_TRG2_ACCBRST_seq2=Burst - not interruptible  ADC1_NINSEL_seq2_TXT=Vss - single ended (unsigned)  ADC2_NINSEL_seq2_TXT=Vss - single ended (unsigned)  ADC3_NINSEL_seq2_TXT=Vss - single ended (unsigned)  ADC4_NINSEL_seq2_TXT=Vss - single ended (unsigned)  ADC5_NINSEL_seq2_TXT=Vss - single ended (unsigned)  TrigTimeStep_seq2=off  info_seq2=0  TrigSource_seq3_TXT=after previous sequence  SampleTime_seq3_Tad_TXT="0.5 Tad  = 6.25ns  -  Rin < 0 kOhm"  ADC1_seq3_TXT=Not Used  ADC1_seq3_align=Right aligned  ADC1_seq3_overSampling=x1 (12 bits)  ADC2_seq3_TXT=Not Used  ADC2_seq3_align=Right aligned  ADC2_seq3_overSampling=x1 (12 bits)  ADC3_seq3_TXT=Not Used  ADC3_seq3_align=Right aligned  ADC3_seq3_overSampling=x1 (12 bits)  ADC4_seq3_TXT=Not Used  ADC4_seq3_align=Right aligned  ADC4_seq3_overSampling=x1 (12 bits)  ADC5_seq3_TXT=Not Used  ADC5_seq3_align=Right aligned  ADC5_seq3_overSampling=x1 (12 bits)  ADC1_seq3_1_TXT=Not Used  ADC1_seq3_1_align=Right aligned  ADC1_seq3_1_overSampling=x1 (12 bits)  ADC2_seq3_1_TXT=Not Used  ADC2_seq3_1_align=Right aligned  ADC2_seq3_1_overSampling=x1 (12 bits)  ADC3_seq3_1_TXT=Not Used  ADC3_seq3_1_align=Right aligned  ADC3_seq3_1_overSampling=x1 (12 bits)  ADC4_seq3_1_TXT=Not Used  ADC4_seq3_1_align=Right aligned  ADC4_seq3_1_overSampling=x1 (12 bits)  ADC5_seq3_1_TXT=Not Used  ADC5_seq3_1_align=Right aligned  ADC5_seq3_1_overSampling=x1 (12 bits)  ADC1_seq3_2_TXT=Not Used  ADC1_seq3_2_align=Right aligned  ADC1_seq3_2_overSampling=x1 (12 bits)  ADC2_seq3_2_TXT=Not Used  ADC2_seq3_2_align=Right aligned  ADC2_seq3_2_overSampling=x1 (12 bits)  ADC3_seq3_2_TXT=Not Used  ADC3_seq3_2_align=Right aligned  ADC3_seq3_2_overSampling=x1 (12 bits)  ADC4_seq3_2_TXT=Not Used  ADC4_seq3_2_align=Right aligned  ADC4_seq3_2_overSampling=x1 (12 bits)  ADC5_seq3_2_TXT=Not Used  ADC5_seq3_2_align=Right aligned  ADC5_seq3_2_overSampling=x1 (12 bits)  ADC1_seq3_3_TXT=Not Used  ADC1_seq3_3_align=Right aligned  ADC1_seq3_3_overSampling=x1 (12 bits)  ADC2_seq3_3_TXT=Not Used  ADC2_seq3_3_align=Right aligned  ADC2_seq3_3_overSampling=x1 (12 bits)  ADC3_seq3_3_TXT=Not Used  ADC3_seq3_3_align=Right aligned  ADC3_seq3_3_overSampling=x1 (12 bits)  ADC4_seq3_3_TXT=Not Used  ADC4_seq3_3_align=Right aligned  ADC4_seq3_3_overSampling=x1 (12 bits)  ADC5_seq3_3_TXT=Not Used  ADC5_seq3_3_align=Right aligned  ADC5_seq3_3_overSampling=x1 (12 bits)  ADC1_seq3_4_TXT=Not Used  ADC1_seq3_4_align=Right aligned  ADC1_seq3_4_overSampling=x1 (12 bits)  ADC2_seq3_4_TXT=Not Used  ADC2_seq3_4_align=Right aligned  ADC2_seq3_4_overSampling=x1 (12 bits)  ADC3_seq3_4_TXT=Not Used  ADC3_seq3_4_align=Right aligned  ADC3_seq3_4_overSampling=x1 (12 bits)  ADC4_seq3_4_TXT=Not Used  ADC4_seq3_4_align=Right aligned  ADC4_seq3_4_overSampling=x1 (12 bits)  ADC5_seq3_4_TXT=Not Used  ADC5_seq3_4_align=Right aligned  ADC5_seq3_4_overSampling=x1 (12 bits)  ADC1_seq3_5_TXT=Not Used  ADC1_seq3_5_align=Right aligned  ADC1_seq3_5_overSampling=x1 (12 bits)  ADC2_seq3_5_TXT=Not Used  ADC2_seq3_5_align=Right aligned  ADC2_seq3_5_overSampling=x1 (12 bits)  ADC3_seq3_5_TXT=Not Used  ADC3_seq3_5_align=Right aligned  ADC3_seq3_5_overSampling=x1 (12 bits)  ADC4_seq3_5_TXT=Not Used  ADC4_seq3_5_align=Right aligned  ADC4_seq3_5_overSampling=x1 (12 bits)  ADC5_seq3_5_TXT=Not Used  ADC5_seq3_5_align=Right aligned  ADC5_seq3_5_overSampling=x1 (12 bits)  ADC_TRG2_ACCBRST_seq3=Burst - not interruptible  ADC1_NINSEL_seq3_TXT=Vss - single ended (unsigned)  ADC2_NINSEL_seq3_TXT=Vss - single ended (unsigned)  ADC3_NINSEL_seq3_TXT=Vss - single ended (unsigned)  ADC4_NINSEL_seq3_TXT=Vss - single ended (unsigned)  ADC5_NINSEL_seq3_TXT=Vss - single ended (unsigned)  TrigTimeStep_seq3=off  info_seq3=0  TrigSource_seq4_TXT=after previous sequence  SampleTime_seq4_Tad_TXT="0.5 Tad  = 6.25ns  -  Rin < 0 kOhm"  ADC1_seq4_TXT=Not Used  ADC1_seq4_align=Right aligned  ADC1_seq4_overSampling=x1 (12 bits)  ADC2_seq4_TXT=Not Used  ADC2_seq4_align=Right aligned  ADC2_seq4_overSampling=x1 (12 bits)  ADC3_seq4_TXT=Not Used  ADC3_seq4_align=Right aligned  ADC3_seq4_overSampling=x1 (12 bits)  ADC4_seq4_TXT=Not Used  ADC4_seq4_align=Right aligned  ADC4_seq4_overSampling=x1 (12 bits)  ADC5_seq4_TXT=Not Used  ADC5_seq4_align=Right aligned  ADC5_seq4_overSampling=x1 (12 bits)  ADC1_seq4_1_TXT=Not Used  ADC1_seq4_1_align=Right aligned  ADC1_seq4_1_overSampling=x1 (12 bits)  ADC2_seq4_1_TXT=Not Used  ADC2_seq4_1_align=Right aligned  ADC2_seq4_1_overSampling=x1 (12 bits)  ADC3_seq4_1_TXT=Not Used  ADC3_seq4_1_align=Right aligned  ADC3_seq4_1_overSampling=x1 (12 bits)  ADC4_seq4_1_TXT=Not Used  ADC4_seq4_1_align=Right aligned  ADC4_seq4_1_overSampling=x1 (12 bits)  ADC5_seq4_1_TXT=Not Used  ADC5_seq4_1_align=Right aligned  ADC5_seq4_1_overSampling=x1 (12 bits)  ADC1_seq4_2_TXT=Not Used  ADC1_seq4_2_align=Right aligned  ADC1_seq4_2_overSampling=x1 (12 bits)  ADC2_seq4_2_TXT=Not Used  ADC2_seq4_2_align=Right aligned  ADC2_seq4_2_overSampling=x1 (12 bits)  ADC3_seq4_2_TXT=Not Used  ADC3_seq4_2_align=Right aligned  ADC3_seq4_2_overSampling=x1 (12 bits)  ADC4_seq4_2_TXT=Not Used  ADC4_seq4_2_align=Right aligned  ADC4_seq4_2_overSampling=x1 (12 bits)  ADC5_seq4_2_TXT=Not Used  ADC5_seq4_2_align=Right aligned  ADC5_seq4_2_overSampling=x1 (12 bits)  ADC1_seq4_3_TXT=Not Used  ADC1_seq4_3_align=Right aligned  ADC1_seq4_3_overSampling=x1 (12 bits)  ADC2_seq4_3_TXT=Not Used  ADC2_seq4_3_align=Right aligned  ADC2_seq4_3_overSampling=x1 (12 bits)  ADC3_seq4_3_TXT=Not Used  ADC3_seq4_3_align=Right aligned  ADC3_seq4_3_overSampling=x1 (12 bits)  ADC4_seq4_3_TXT=Not Used  ADC4_seq4_3_align=Right aligned  ADC4_seq4_3_overSampling=x1 (12 bits)  ADC5_seq4_3_TXT=Not Used  ADC5_seq4_3_align=Right aligned  ADC5_seq4_3_overSampling=x1 (12 bits)  ADC1_seq4_4_TXT=Not Used  ADC1_seq4_4_align=Right aligned  ADC1_seq4_4_overSampling=x1 (12 bits)  ADC2_seq4_4_TXT=Not Used  ADC2_seq4_4_align=Right aligned  ADC2_seq4_4_overSampling=x1 (12 bits)  ADC3_seq4_4_TXT=Not Used  ADC3_seq4_4_align=Right aligned  ADC3_seq4_4_overSampling=x1 (12 bits)  ADC4_seq4_4_TXT=Not Used  ADC4_seq4_4_align=Right aligned  ADC4_seq4_4_overSampling=x1 (12 bits)  ADC5_seq4_4_TXT=Not Used  ADC5_seq4_4_align=Right aligned  ADC5_seq4_4_overSampling=x1 (12 bits)  ADC1_seq4_5_TXT=Not Used  ADC1_seq4_5_align=Right aligned  ADC1_seq4_5_overSampling=x1 (12 bits)  ADC2_seq4_5_TXT=Not Used  ADC2_seq4_5_align=Right aligned  ADC2_seq4_5_overSampling=x1 (12 bits)  ADC3_seq4_5_TXT=Not Used  ADC3_seq4_5_align=Right aligned  ADC3_seq4_5_overSampling=x1 (12 bits)  ADC4_seq4_5_TXT=Not Used  ADC4_seq4_5_align=Right aligned  ADC4_seq4_5_overSampling=x1 (12 bits)  ADC5_seq4_5_TXT=Not Used  ADC5_seq4_5_align=Right aligned  ADC5_seq4_5_overSampling=x1 (12 bits)  ADC_TRG2_ACCBRST_seq4=Burst - not interruptible  ADC1_NINSEL_seq4_TXT=Vss - single ended (unsigned)  ADC2_NINSEL_seq4_TXT=Vss - single ended (unsigned)  ADC3_NINSEL_seq4_TXT=Vss - single ended (unsigned)  ADC4_NINSEL_seq4_TXT=Vss - single ended (unsigned)  ADC5_NINSEL_seq4_TXT=Vss - single ended (unsigned)  TrigTimeStep_seq4=off  info_seq4=0  TrigSource_seq5_TXT=after previous sequence  SampleTime_seq5_Tad_TXT="0.5 Tad  = 6.25ns  -  Rin < 0 kOhm"  ADC1_seq5_TXT=Not Used  ADC1_seq5_align=Right aligned  ADC1_seq5_overSampling=x1 (12 bits)  ADC2_seq5_TXT=Not Used  ADC2_seq5_align=Right aligned  ADC2_seq5_overSampling=x1 (12 bits)  ADC3_seq5_TXT=Not Used  ADC3_seq5_align=Right aligned  ADC3_seq5_overSampling=x1 (12 bits)  ADC4_seq5_TXT=Not Used  ADC4_seq5_align=Right aligned  ADC4_seq5_overSampling=x1 (12 bits)  ADC5_seq5_TXT=Not Used  ADC5_seq5_align=Right aligned  ADC5_seq5_overSampling=x1 (12 bits)  ADC1_seq5_1_TXT=Not Used  ADC1_seq5_1_align=Right aligned  ADC1_seq5_1_overSampling=x1 (12 bits)  ADC2_seq5_1_TXT=Not Used  ADC2_seq5_1_align=Right aligned  ADC2_seq5_1_overSampling=x1 (12 bits)  ADC3_seq5_1_TXT=Not Used  ADC3_seq5_1_align=Right aligned  ADC3_seq5_1_overSampling=x1 (12 bits)  ADC4_seq5_1_TXT=Not Used  ADC4_seq5_1_align=Right aligned  ADC4_seq5_1_overSampling=x1 (12 bits)  ADC5_seq5_1_TXT=Not Used  ADC5_seq5_1_align=Right aligned  ADC5_seq5_1_overSampling=x1 (12 bits)  ADC1_seq5_2_TXT=Not Used  ADC1_seq5_2_align=Right aligned  ADC1_seq5_2_overSampling=x1 (12 bits)  ADC2_seq5_2_TXT=Not Used  ADC2_seq5_2_align=Right aligned  ADC2_seq5_2_overSampling=x1 (12 bits)  ADC3_seq5_2_TXT=Not Used  ADC3_seq5_2_align=Right aligned  ADC3_seq5_2_overSampling=x1 (12 bits)  ADC4_seq5_2_TXT=Not Used  ADC4_seq5_2_align=Right aligned  ADC4_seq5_2_overSampling=x1 (12 bits)  ADC5_seq5_2_TXT=Not Used  ADC5_seq5_2_align=Right aligned  ADC5_seq5_2_overSampling=x1 (12 bits)  ADC1_seq5_3_TXT=Not Used  ADC1_seq5_3_align=Right aligned  ADC1_seq5_3_overSampling=x1 (12 bits)  ADC2_seq5_3_TXT=Not Used  ADC2_seq5_3_align=Right aligned  ADC2_seq5_3_overSampling=x1 (12 bits)  ADC3_seq5_3_TXT=Not Used  ADC3_seq5_3_align=Right aligned  ADC3_seq5_3_overSampling=x1 (12 bits)  ADC4_seq5_3_TXT=Not Used  ADC4_seq5_3_align=Right aligned  ADC4_seq5_3_overSampling=x1 (12 bits)  ADC5_seq5_3_TXT=Not Used  ADC5_seq5_3_align=Right aligned  ADC5_seq5_3_overSampling=x1 (12 bits)  ADC1_seq5_4_TXT=Not Used  ADC1_seq5_4_align=Right aligned  ADC1_seq5_4_overSampling=x1 (12 bits)  ADC2_seq5_4_TXT=Not Used  ADC2_seq5_4_align=Right aligned  ADC2_seq5_4_overSampling=x1 (12 bits)  ADC3_seq5_4_TXT=Not Used  ADC3_seq5_4_align=Right aligned  ADC3_seq5_4_overSampling=x1 (12 bits)  ADC4_seq5_4_TXT=Not Used  ADC4_seq5_4_align=Right aligned  ADC4_seq5_4_overSampling=x1 (12 bits)  ADC5_seq5_4_TXT=Not Used  ADC5_seq5_4_align=Right aligned  ADC5_seq5_4_overSampling=x1 (12 bits)  ADC1_seq5_5_TXT=Not Used  ADC1_seq5_5_align=Right aligned  ADC1_seq5_5_overSampling=x1 (12 bits)  ADC2_seq5_5_TXT=Not Used  ADC2_seq5_5_align=Right aligned  ADC2_seq5_5_overSampling=x1 (12 bits)  ADC3_seq5_5_TXT=Not Used  ADC3_seq5_5_align=Right aligned  ADC3_seq5_5_overSampling=x1 (12 bits)  ADC4_seq5_5_TXT=Not Used  ADC4_seq5_5_align=Right aligned  ADC4_seq5_5_overSampling=x1 (12 bits)  ADC5_seq5_5_TXT=Not Used  ADC5_seq5_5_align=Right aligned  ADC5_seq5_5_overSampling=x1 (12 bits)  ADC_TRG2_ACCBRST_seq5=Burst - not interruptible  ADC1_NINSEL_seq5_TXT=Vss - single ended (unsigned)  ADC2_NINSEL_seq5_TXT=Vss - single ended (unsigned)  ADC3_NINSEL_seq5_TXT=Vss - single ended (unsigned)  ADC4_NINSEL_seq5_TXT=Vss - single ended (unsigned)  ADC5_NINSEL_seq5_TXT=Vss - single ended (unsigned)  TrigTimeStep_seq5=off  info_seq5=0
      settings: SourceProductName=MPLAB Device Blocks for Simulink
  Ground : Ground
  QEI1 : MCHP_Blockset/QEI/QEI  QEI_REF=1  QEI_MODE=Quadrature Encoder  QEI_x2mode=off  QEI_PulseCountDir=Down  PIN_QEA_TXT=C6 / P39 / Pin[35]  PIN_QEB_TXT=C7 / P40 / Pin[36]  SWPAB=off  QEAPOL=off  QEBPOL=off  SampleTime=Ts  PIN_CCMP_TXT=A4 / P20 / Pin[33]  MCHP_PORT={QEI1 A}{QEIA1}5:0:P39;{QEI1 B}{QEIB1}5:0:P40;  MCHP_MASTERLINK=MicrochipTargetMotorControl/Microcontroller/HWConfigurations/Microchip Master  INDXxCNT_Output=is not an output  POSxCNT_Output=is a 16 bits unsigned block output  RESET_Input=off  PIMOD_mode=position is cyclique between user defined boundaries  PIMOD_modeB=Never reset position  PIMOD_reset=on next INDEX event  PIN_INDEX_TXT=C8 / P41 / Pin[33]  IMV=QEA = 0 and QEB = 0  IMV_x2=QEA = 1  PIN_HOME_TXT=B0 / P17 / Pin[20]  QEIxLEC_GEC=[0 (65535-1)]  QEIxIC=0  PCIIRQ=off  IDXPOL=on  HOMPOL=on  VELxCNT_Output=is not an output  INTxHLD_Output=is not an output  MaxPeriod=1e-3  FILTREN=on  QFDIV_popup_TXT=520.83 kHz  FILTER_CutOffFreq=100e3  QEI_IntPri=5
      settings: SourceProductName=MPLAB Device Blocks for Simulink
  Terminator{,1..3} (4 alike) : Terminator
  Vector Concatenate : Concatenate
  Vector Concatenate1 : Concatenate
  Vector Concatenate2 : Concatenate  NumInputs=3
  IabADC : Outport
  VdcADC : Outport  Port=2
  VabcADC : Outport  Port=3
  eQEP : Outport  Port=4
  wires:
  Vector Concatenate/1 -> IabADC/1
  ADC HS 12b dsPICA1/2 -> Vector Concatenate/2
  ADC HS 12b dsPICA1/1 -> Vector Concatenate/1
  PhaseCurrFb/1 -> Terminator/1
  PositionFb/1 -> Terminator1/1
  QEI1/1 -> Vector Concatenate1/1  "theta_RAW"
  Vector Concatenate1/1 -> eQEP/1
  Vector Concatenate2/1 -> VabcADC/1
  ADC HS 12b dsPICA1/3 -> Vector Concatenate2/2
  ADC HS 12b dsPICA1/5 -> Vector Concatenate2/3
  ADC HS 12b dsPICA2/3 -> Terminator3/1
  ADC HS 12b dsPICA2/2 -> VdcADC/1
  ADC HS 12b dsPICA2/1 -> Terminator2/1
  ADC HS 12b dsPICA1/4 -> Vector Concatenate2/1
  Ground/1 -> Vector Concatenate1/2

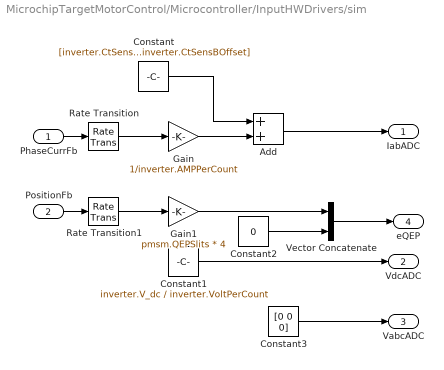
== system MicrochipTargetMotorControl/Microcontroller/InputHWDrivers/sim ==
  PhaseCurrFb : Inport
  PositionFb : Inport  Port=2
  Add : Sum  RndMeth=Simplest  OutDataTypeStr=Inherit: Same as first input
  Constant : Constant  Value=[inverter.CtSensAOffset inverter.CtSensBOffset]  OutDataTypeStr=int16
  Constant1 : Constant  Value=inverter.V_dc / inverter.VoltPerCount  OutDataTypeStr=uint16  SampleTime=Ts
  Constant2 : Constant  Value=0  OutDataTypeStr=Inherit: Inherit via back propagation  SampleTime=Ts
  Constant3 : Constant  Value=[0 0 0]  OutDataTypeStr=uint16  SampleTime=Ts
  Gain : Gain  Gain=1/inverter.AMPPerCount  OutDataTypeStr=int16  RndMeth=Simplest
  Gain1 : Gain  Gain=pmsm.QEPSlits * 4  OutDataTypeStr=uint16  RndMeth=Simplest
  Rate Transition : RateTransition  Deterministic=off  OutPortSampleTime=Ts
  Rate Transition1 : RateTransition  Deterministic=off  OutPortSampleTime=Ts
  Vector Concatenate : Concatenate
  IabADC : Outport
  VdcADC : Outport  Port=2
  VabcADC : Outport  Port=3
  eQEP : Outport  Port=4
  wires:
  PhaseCurrFb/1 -> Rate Transition/1
  Gain/1 -> Add/2
  Constant/1 -> Add/1
  Add/1 -> IabADC/1
  PositionFb/1 -> Rate Transition1/1
  Gain1/1 -> Vector Concatenate/1
  Constant1/1 -> VdcADC/1
  Vector Concatenate/1 -> eQEP/1
  Constant2/1 -> Vector Concatenate/2
  Rate Transition/1 -> Gain/1
  Rate Transition1/1 -> Gain1/1
  Constant3/1 -> VabcADC/1

== system MicrochipTargetMotorControl/Microcontroller/InputScaling/Calculate phase currents ==
  Mode : Inport
  Iab_ADC : Inport  Port=2
  Automatic offset calibration : Subsystem  VariantControl=inverter.ADCOffsetCalibEnable == 1
  Offser via parameter : Subsystem  VariantControl=inverter.ADCOffsetCalibEnable == 0
  Iabc : Outport

== system MicrochipTargetMotorControl/Microcontroller/ModeControl/ClosedLoop ==
  Constant : Constant  Value=2  OutDataTypeStr=single  SampleTime=0.1
  Mode : Outport
  wires:
  Constant/1 -> Mode/1

== system MicrochipTargetMotorControl/Microcontroller/ModeControl/CurrentCalib ==
  Step : Step  After=2  OutDataTypeStr=single  SampleTime=0.1
  Mode : Outport
  wires:
  Step/1 -> Mode/1

== system MicrochipTargetMotorControl/Microcontroller/ModeControl/CurrentPosCalib ==
  Add : Sum
  Step : Step  OutDataTypeStr=single  SampleTime=0.1
  Step1 : Step  Time=2  OutDataTypeStr=single  SampleTime=0.1
  Mode : Outport
  wires:
  Step/1 -> Add/1
  Step1/1 -> Add/2
  Add/1 -> Mode/1

== system MicrochipTargetMotorControl/Microcontroller/ModeControl/PosCalib ==
  Step : Step  Before=1  After=2  OutDataTypeStr=single  SampleTime=0.1
  Mode : Outport
  wires:
  Step/1 -> Mode/1
